simulink model "Mosaic_Motion__TestBench"  (R2025b)
settings: Solver=FixedStepAuto  StartTime=0.0  StopTime=1000  FixedStep=dt  RelTol=1e-3
undefined symbols (not defined in the file): J_pitch, J_yaw, pitchMot, yawMot
libraries: simulink_extras x4, Simscape_Gimbals__Lib x3, dspstat3 x2
settings Model: Creator=Leonid  LastModifiedBy=Leonid

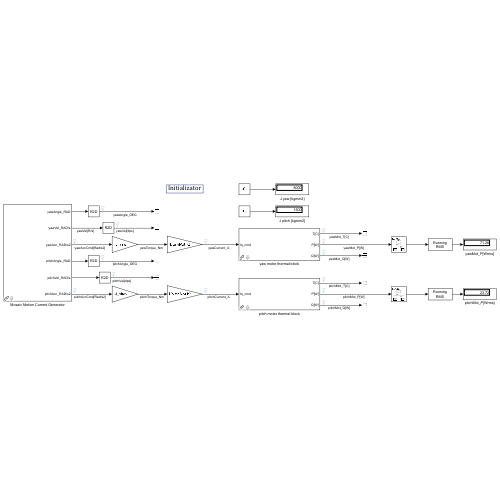
[thumbnail: Simulink's stored preview of the top-level diagram]
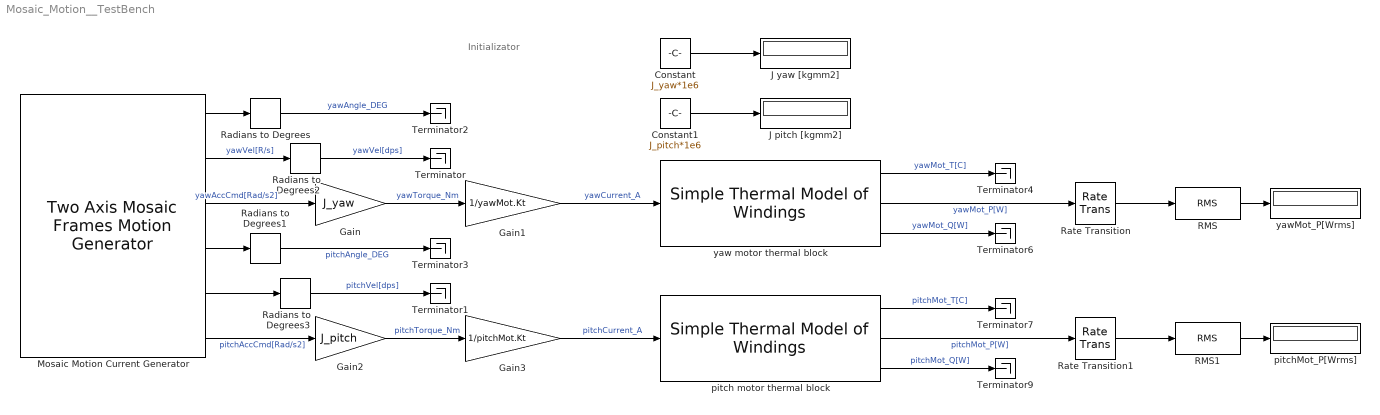
== system Mosaic_Motion__TestBench ==
  note: Initializator
  Constant : Constant  Value=J_yaw*1e6
  Constant1 : Constant  Value=J_pitch*1e6
  Gain : Gain  Gain=J_yaw
  Gain1 : Gain  Gain=1/yawMot.Kt
  Gain2 : Gain  Gain=J_pitch
  Gain3 : Gain  Gain=1/pitchMot.Kt
  J pitch [kgmm2] : Display
  J yaw [kgmm2] : Display
  Mosaic Motion Current Generator : Simscape_Gimbals__Lib/Two Axis Mosaic Frames Motion Generator  dt=dt  tFrame=tFrame  tMotion=tMotion  nFrames=nFrames  yawVec_DEG=yawVec  pitchVec_DEG=pitchVec
  RMS : dspstat3/RMS  run=on  directionMode=Entire input  dimension=1  reset_popup=None
  RMS1 : dspstat3/RMS  run=on  directionMode=Entire input  dimension=1  reset_popup=None
  Radians to Degrees{,1..3} (4 alike) : simulink_extras/Transformations/Radians to Degrees
  Rate Transition : RateTransition  OutPortSampleTime=dt
  Rate Transition1 : RateTransition  OutPortSampleTime=dt
  Terminator{,1..4,6..7,9} (8 alike) : Terminator
  pitch motor thermal block : Simscape_Gimbals__Lib/Simple Thermal Model of Windings  T_env=Tenv  T_ini=Tini  wind_m=pitchMot.m  wind_R=pitchMot.R  wind_Rth=pitchMot.Rth*0.7
  pitchMot_P[Wrms] : Display
      settings: Decimation=5
  yaw motor thermal block : Simscape_Gimbals__Lib/Simple Thermal Model of Windings  T_env=Tenv  T_ini=Tini  wind_m=yawMot.m  wind_R=yawMot.R  wind_Rth=yawMot.Rth*0.7
  yawMot_P[Wrms] : Display
  wires:
  Mosaic Motion Current Generator/1 -> Radians to Degrees/1
  Mosaic Motion Current Generator/2 -> Radians to Degrees2/1  "yawVel[R/s]"
  Mosaic Motion Current Generator/4 -> Radians to Degrees1/1
  Mosaic Motion Current Generator/3 -> Gain/1  "yawAccCmd[Rad/s2]"
  Radians to Degrees/1 -> Terminator2/1  "yawAngle_DEG"
  Radians to Degrees1/1 -> Terminator3/1  "pitchAngle_DEG"
  Mosaic Motion Current Generator/5 -> Radians to Degrees3/1
  Gain/1 -> Gain1/1  "yawTorque_Nm"
  Gain1/1 -> yaw motor thermal block/1  "yawCurrent_A"
  Mosaic Motion Current Generator/6 -> Gain2/1  "pitchAccCmd[Rad/s2]"
  Gain2/1 -> Gain3/1  "pitchTorque_Nm"
  Gain3/1 -> pitch motor thermal block/1  "pitchCurrent_A"
  yaw motor thermal block/1 -> Terminator4/1  "yawMot_T[C]"
  yaw motor thermal block/2 -> Rate Transition/1  "yawMot_P[W]"
  yaw motor thermal block/3 -> Terminator6/1  "yawMot_Q[W]"
  pitch motor thermal block/1 -> Terminator7/1  "pitchMot_T[C]"
  pitch motor thermal block/2 -> Rate Transition1/1  "pitchMot_P[W]"
  pitch motor thermal block/3 -> Terminator9/1  "pitchMot_Q[W]"
  Radians to Degrees2/1 -> Terminator/1  "yawVel[dps]"
  Radians to Degrees3/1 -> Terminator1/1  "pitchVel[dps]"
  Constant/1 -> J yaw [kgmm2]/1
  Constant1/1 -> J pitch [kgmm2]/1
  RMS/1 -> yawMot_P[Wrms]/1
  RMS1/1 -> pitchMot_P[Wrms]/1
  Rate Transition/1 -> RMS/1
  Rate Transition1/1 -> RMS1/1
